simulink model "MSE452_Lab4_grid_side_VOC_student"  (R2023a)
settings: Solver=ode23tb  StartTime=0.0  StopTime=1  MaxStep=1e-5  RelTol=1e-5  AbsTol=1e-5  EnableMultiTasking=on
values from neighbouring files (symbols this model uses):
  Cdc = 4*Cb    [MSE452_Lab4_grid_side_VOC.m]
  Fb = 60    [MSE452_Lab4_grid_side_VOC.m]
  Fs = 2040    [MSE452_Lab4_grid_side_VOC.m]
  Fsampling = 10e3    (= 10000)    [MSE452_Lab4_grid_side_VOC.m]
  Ib = Pb/(Vb)    [MSE452_Lab4_grid_side_VOC.m]
  Lgrid = Lgrid_pu*Lb    [MSE452_Lab4_grid_side_VOC.m]
  Lgrid_pu = 0.2    [MSE452_Lab4_grid_side_VOC.m]
  Rdc_series = 0.1*Zb    [MSE452_Lab4_grid_side_VOC.m]
  Rgrid = Rgrid_pu*Zb    [MSE452_Lab4_grid_side_VOC.m]
  Vb = 690/sqrt(3)    [MSE452_Lab4_grid_side_VOC.m]
  Vdc_ref = sqrt(6)*(1/0.8)    [MSE452_Lab4_grid_side_VOC.m]
  Vdc_supply = Vdc_ref*Vb + Idc*Rdc_series    [MSE452_Lab4_grid_side_VOC.m]
undefined symbols (not defined in the file or in its folder): Rdc
libraries: spsVoltageMeasurementLib x4, spsCurrentMeasurementLib x3, powerlib_extras x3, simulink x3, spsSeriesRLCBranchLib x2, spsControlledVoltageSourceLib x2, simulink_extras x2, spsDCVoltageSourceLib x1, spsUniversalBridgeLib x1, spsThreePhaseSeriesRLCBranchLib x1, spsPower3phInstantaneousLib x1, sps_lib x1
settings Model: Creator=lang  LastModifiedBy=auamai
settings SolverCC: AutoScaleAbsTol=off  AlgebraicLoopSolver=TrustRegion
settings DataIOCC: LimitDataPoints=on  SaveFormat=Array  SignalLoggingSaveFormat=ModelDataLogs  ReturnWorkspaceOutputs=off
settings OptimizationCC: ExpressionDepthLimit=2147483647  InitFltsAndDblsToZero=on  LifeSpan=inf
settings DebuggingCC: SaveWithParameterizedLinksMsg=none  UnderspecifiedInitializationDetection=Classic  MergeDetectMultiDrivingBlocksExec=none  SolverPrmCheckMsg=warning  MultiTaskCondExecSysMsg=none  FcnCallInpInsideContextMsg=warning  UnconnectedInputMsg=warning  UnconnectedOutputMsg=warning  UnconnectedLineMsg=warning  StateNameClashWarn=warning  SFUnexpectedBacktrackingDiag=warning  SFNoUnconditionalDefaultTransitionDiag=warning  SFExecutionAtInitializationDiag=none  ArithmeticOperatorsInVariantConditions=warning
settings HardwareCC: ProdBitPerPointer=32  ProdBitPerSizeT=32  ProdBitPerPtrDiffT=32  ProdLargestAtomicFloat=None  ProdIntDivRoundTo=Undefined  ProdEndianess=Unspecified  ProdWordSize=32  ProdHWDeviceType=32-bit Generic
settings ModelReferenceCC: EnableRefExpFcnMdlSchedulingChecks=on  PropagateSignalLabelsOutOfModel=off
settings SFSimCC: SimUseLocalCustomCode=off  SimParseCustomCode=off  CustomCodeUndefinedFunction=UseInterfaceOnly
settings RTWCC: RTWUseLocalCustomCode=off
settings CodeAppCC: StateflowObjectComments=on
settings GRTTargetCC: TargetFcnLib=ansi_tfl_tmw.mat  TargetLangStandard=C89/C90 (ANSI)  CombineOutputUpdateFcns=off  GRTInterface=on
settings ConfigComp: CovMetricSettings=dw  CovSaveCumulativeToWorkspaceVar=on  CovSaveSingleToWorkspaceVar=on  CovExternalEMLEnable=off
settings SimscapeCC: SimscapeNormalizeSystem=off

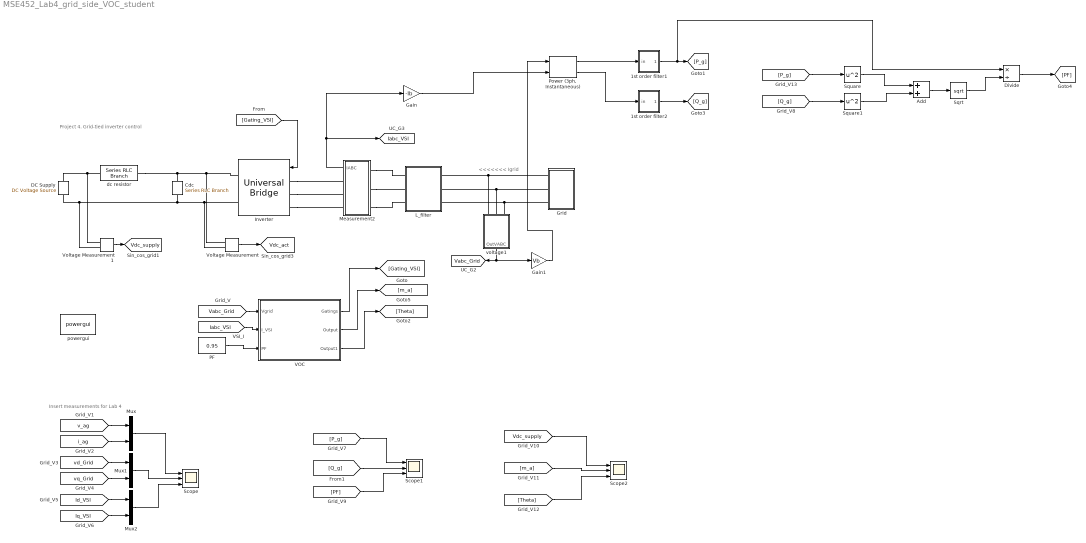
== system MSE452_Lab4_grid_side_VOC_student ==
  note: Insert measurements for Lab 4
  note: <<<<<<< Igrid
  note: Project 4. Grid-tied inverter control
  " voltage1" : Subsystem  mask{Base=Vb}
      mask prompts: Base "Base value"
  1st order filter1 : Subsystem  mask{F0=10, Fs=Fsampling}
      mask prompts: F0 "Cut off Frequency"; Fs "Sampling Frequency"
  1st order filter2 : Subsystem  mask{F0=10, Fs=Fsampling}
      mask prompts: F0 "Cut off Frequency"; Fs "Sampling Frequency"
  Add : Sum
  Cdc : spsSeriesRLCBranchLib/Series RLC Branch  LConnTagsString=__new0  RConnTagsString=__new0  BranchType=C  Resistance=Rdc  Inductance=1e-3  SetiL0=off  InitialCurrent=0  Capacitance=Cdc  Setx0=on  InitialVoltage=Vdc_capacitor_initial  Measurements=None
  DC Supply : spsDCVoltageSourceLib/DC Voltage Source  Amplitude=Vdc_supply*1.0  Measurements=None
  Divide : Product  Inputs=*/
  Gain : Gain  Gain=-Ib
  Gain1 : Gain  Gain=Vb
  Grid : Subsystem
  Inverter : spsUniversalBridgeLib/Universal Bridge  Arms=3  SnubberResistance=1e5  SnubberCapacitance=inf  Device=IGBT / Diodes  Ron=1e-6  Lon=0  ForwardVoltages="[  0  0  ]"  ForwardVoltage=0  GTOparameters=[ 10e-6 , 20e-6 ]  IGBTparameters=[ 1e-6 , 2e-6 ]  Measurements=None  Measurements_2=None  converterType=Rectifier
  L_filter : Subsystem
  Measurement2 : Subsystem  mask{Base=Ib}
      mask prompts: Base "Base value"
  Mux : Mux  Inputs=2
  Mux1 : Mux  Inputs=2
  Mux2 : Mux  Inputs=2
  PF : Constant  Value=0.95
  "Power (3ph, Instantaneous)" : spsPower3phInstantaneousLib/Power (3ph, Instantaneous)
  Scope : Scope  NumInputPorts=3
  Scope1 : Scope  NumInputPorts=3
  Scope2 : Scope  NumInputPorts=3
  Sqrt : Sqrt
  Square : Math  Operator=square
  Square1 : Math  Operator=square
  VOC : Subsystem
  Voltage Measurement : spsVoltageMeasurementLib/Voltage Measurement  PhasorSimulation=off  OutputType=Complex  PSBequivalent=0
  Voltage Measurement1 : spsVoltageMeasurementLib/Voltage Measurement  PhasorSimulation=off  OutputType=Complex  PSBequivalent=0
  dc resistor : spsSeriesRLCBranchLib/Series RLC Branch  LConnTagsString=__new0  RConnTagsString=__new0  BranchType=R  Resistance=Rdc_series  Inductance=1e-3  SetiL0=off  InitialCurrent=0  Capacitance=1e-6  Setx0=off  InitialVoltage=0  Measurements=None
  powergui : sps_lib/powergui  Priority=1  SimulationMode=Continuous  SampleTime=50e-6  frequency=60  Iterations=50  frequencyindice=0  Pbase=100e6  ErrMax=1e-4  UnitsV=kV  UnitsW=MW  buscounter=0  FunctionMessages=off  echomessages=off  EnableUseOfTLC=off  CurrentSourceSwitches=on  DisableSnubberDevices=off  DisableRonSwitches=off  DisableVfSwitches=off  DisplayEquations=off  AutomaticDiscreteSolvers=off  SolverType=Tustin  Interpol=off  ExternalGateDelay=off  methode=off  Ts=100  x0status=blocks  SPID=off  SwTol=0  HookPort=off  NonlinearTolerance=1e-4  nMaxIteration=100  ContinueOnMaxIteration=off  RestoreLinks=warning  ResistiveCurrentMeasurement=off  Frange=[0:2:500]  Ylog=off  Xlog=on  ShowGrid=off  save=off  variable=ZData  structure=0  ZoomFFT=off  StartTime=0.0  cycles=1  DisplayStyle=1  fundamental=60  FreqAxis=off  MaxFrequency=1000  frequencyindicesteady=1  RmsSteady=1  display=off
  tag scope: Iabc_VSI=global, Vabc_Grid=global, Vdc_act=global, Vdc_supply=global
  wires:
  [Vabc_Grid] -> VOC/1(Vgrid)
  [Iabc_VSI] -> VOC/2(I_VSI)
  VOC/1(Gatings) -> [Gating_VSI]
  [Gating_VSI] -> Inverter/1
  Voltage Measurement/1 -> [Vdc_act]
  Voltage Measurement1/1 -> [Vdc_supply]
  Measurement2/1(IABC) -> Gain/1, [Iabc_VSI]
  " voltage1"/1(OutVABC) -> Gain1/1, [Vabc_Grid]
  [v_ag] -> Mux/1
  [i_ag] -> Mux/2
  [vq_Grid] -> Mux1/2
  [vd_Grid] -> Mux1/1
  [Id_VSI] -> Mux2/1
  [Iq_VSI] -> Mux2/2
  PF/1 -> VOC/3(PF)
  Mux/1 -> Scope/1
  Mux1/1 -> Scope/2
  Mux2/1 -> Scope/3
  [P_g] -> Scope1/1
  [Q_g] -> Scope1/2
  [PF] -> Scope1/3
  [Vdc_supply] -> Scope2/1
  [m_a] -> Scope2/2
  [Theta] -> Scope2/3
  VOC/2(Output) -> [m_a]
  VOC/3(Output1) -> [Theta]
  Gain/1 -> "Power (3ph, Instantaneous)"/2
  Gain1/1 -> "Power (3ph, Instantaneous)"/1
  "Power (3ph, Instantaneous)"/1 -> 1st order filter1/1(in)
  "Power (3ph, Instantaneous)"/2 -> 1st order filter2/1(in)
  1st order filter1/1(Out) -> Divide/1, [P_g]
  1st order filter2/1(Out) -> [Q_g]
  [P_g] -> Square/1
  [Q_g] -> Square1/1
  Square/1 -> Add/1
  Square1/1 -> Add/2
  Add/1 -> Sqrt/1
  Sqrt/1 -> Divide/2
  Divide/1 -> [PF]
  connections:
  Cdc/RConn1 -- Voltage Measurement/LConn1 -- Inverter/RConn1 -- dc resistor/RConn1
  Inverter/RConn2 -- Voltage Measurement/LConn2 -- Cdc/LConn1 -- DC Supply/LConn1 -- Voltage Measurement1/LConn2
  DC Supply/RConn1 -- dc resistor/LConn1 -- Voltage Measurement1/LConn1
  Inverter/LConn1 -- Measurement2/RConn1
  Inverter/LConn2 -- Measurement2/RConn2
  Inverter/LConn3 -- Measurement2/RConn3
  Measurement2/LConn1 -- L_filter/RConn1
  Measurement2/LConn2 -- L_filter/RConn2
  Measurement2/LConn3 -- L_filter/RConn3
  " voltage1"/LConn1 -- Grid/RConn1 -- L_filter/LConn1
  " voltage1"/LConn2 -- Grid/RConn2 -- L_filter/LConn2
  " voltage1"/LConn3 -- Grid/RConn3 -- L_filter/LConn3

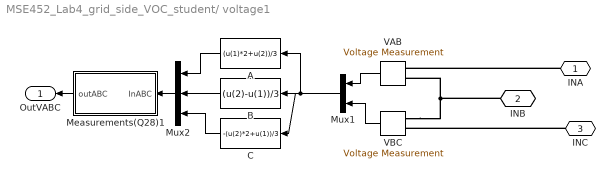
== system MSE452_Lab4_grid_side_VOC_student/ voltage1 ==
  A : Fcn  Expr=(u(1)*2+u(2))/3
  B : Fcn  Expr=(u(2)-u(1))/3
  C : Fcn  Expr=-(u(2)*2+u(1))/3
  Measurements(Q28)1 : Subsystem  mask{Base=Base}
      mask prompts: Base "Base Value"
  Mux1 : Mux  Inputs=2
  Mux2 : Mux  Inputs=3
  VAB : spsVoltageMeasurementLib/Voltage Measurement  PhasorSimulation=off  OutputType=Complex  PSBequivalent=0
  VBC : spsVoltageMeasurementLib/Voltage Measurement  PhasorSimulation=off  OutputType=Complex  PSBequivalent=0
  INA : PMIOPort  Side=Left
  INB : PMIOPort  Port=2  Side=Left
  INC : PMIOPort  Port=3  Side=Left
  OutVABC : Outport
  wires:
  Measurements(Q28)1/1(outABC) -> OutVABC/1
  VAB/1 -> Mux1/1
  VBC/1 -> Mux1/2
  Mux1/1 -> A/1, B/1, C/1
  A/1 -> Mux2/1
  B/1 -> Mux2/2
  Mux2/1 -> Measurements(Q28)1/1(InABC)
  C/1 -> Mux2/3
  connections:
  VBC/LConn1 -- VAB/LConn2 -- INB/RConn1
  INC/RConn1 -- VBC/LConn2
  INA/RConn1 -- VAB/LConn1

== system MSE452_Lab4_grid_side_VOC_student/1st order filter1 ==
  in : Inport
  Discrete Transfer 1Hz3 : DiscreteTransferFcn  Numerator=[1/Fs*(2*pi*F0) 1/Fs*(2*pi*F0) ]  Denominator="[((2*pi*F0)/Fs+2)  ((2*pi*F0)/Fs-2)]"  SampleTime=1/Fs
  Out : Outport
  wires:
  in/1 -> Discrete Transfer 1Hz3/1
  Discrete Transfer 1Hz3/1 -> Out/1

== system MSE452_Lab4_grid_side_VOC_student/1st order filter2 ==
  in : Inport
  Discrete Transfer 1Hz3 : DiscreteTransferFcn  Numerator=[1/Fs*(2*pi*F0) 1/Fs*(2*pi*F0) ]  Denominator="[((2*pi*F0)/Fs+2)  ((2*pi*F0)/Fs-2)]"  SampleTime=1/Fs
  Out : Outport
  wires:
  Discrete Transfer 1Hz3/1 -> Out/1
  in/1 -> Discrete Transfer 1Hz3/1

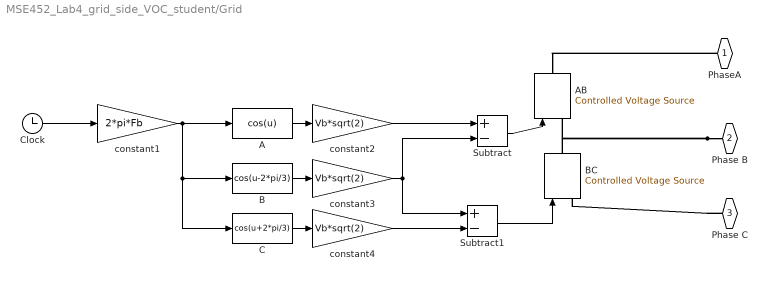
== system MSE452_Lab4_grid_side_VOC_student/Grid ==
  A : Fcn  Expr=cos(u)
  AB : spsControlledVoltageSourceLib/Controlled Voltage Source  Initialize=off  Source_Type=AC  Amplitude=0  Phase=0  Frequency=0  Measurements=None
  B : Fcn  Expr=cos(u-2*pi/3)
  BC : spsControlledVoltageSourceLib/Controlled Voltage Source  Initialize=off  Source_Type=AC  Amplitude=0  Phase=0  Frequency=0  Measurements=None
  C : Fcn  Expr=cos(u+2*pi/3)
  Clock : Clock
  Subtract : Sum  Inputs=+-
  Subtract1 : Sum  Inputs=+-
  constant1 : Gain  Gain=2*pi*Fb
  constant2 : Gain  Gain=Vb*sqrt(2)
  constant3 : Gain  Gain=Vb*sqrt(2)
  constant4 : Gain  Gain=Vb*sqrt(2)
  PhaseA : PMIOPort  Side=Right
  Phase B : PMIOPort  Port=2  Side=Right
  Phase C : PMIOPort  Port=3  Side=Right
  wires:
  Subtract/1 -> AB/1
  Subtract1/1 -> BC/1
  A/1 -> constant2/1
  B/1 -> constant3/1
  C/1 -> constant4/1
  Clock/1 -> constant1/1
  constant1/1 -> A/1, B/1, C/1
  constant2/1 -> Subtract/1
  constant3/1 -> Subtract/2, Subtract1/1
  constant4/1 -> Subtract1/2
  connections:
  Phase B/RConn1 -- BC/RConn1 -- AB/LConn1
  PhaseA/RConn1 -- AB/RConn1
  Phase C/RConn1 -- BC/LConn1

== system MSE452_Lab4_grid_side_VOC_student/L_filter ==
  Three-Phase Series RLC Branch1 : spsThreePhaseSeriesRLCBranchLib/Three-Phase Series RLC Branch  LConnTagsString=A|B|C  RConnTagsString=A|B|C  BranchType=RL  Resistance=Rgrid  Inductance=Lgrid  Capacitance=1e-6  Measurements=None
  In_A : PMIOPort  Side=Left
  out_A : PMIOPort  Port=2  Side=Right
  In_B : PMIOPort  Port=3  Side=Left
  out_B : PMIOPort  Port=4  Side=Right
  In_C : PMIOPort  Port=5  Side=Left
  out_C : PMIOPort  Port=6  Side=Right
  connections:
  In_B/RConn1 -- Three-Phase Series RLC Branch1/LConn2
  out_C/RConn1 -- Three-Phase Series RLC Branch1/RConn3
  out_B/RConn1 -- Three-Phase Series RLC Branch1/RConn2
  out_A/RConn1 -- Three-Phase Series RLC Branch1/RConn1
  Three-Phase Series RLC Branch1/LConn1 -- In_A/RConn1
  Three-Phase Series RLC Branch1/LConn3 -- In_C/RConn1

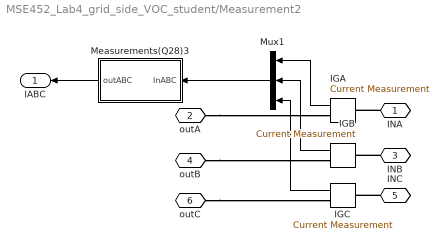
== system MSE452_Lab4_grid_side_VOC_student/Measurement2 ==
  IGA : spsCurrentMeasurementLib/Current Measurement  PhasorSimulation=off  OutputType=Complex  PSBequivalent=0
  IGB : spsCurrentMeasurementLib/Current Measurement  PhasorSimulation=off  OutputType=Complex  PSBequivalent=0
  IGC : spsCurrentMeasurementLib/Current Measurement  PhasorSimulation=off  OutputType=Complex  PSBequivalent=0
  Measurements(Q28)3 : Subsystem  mask{Base=Base}
      mask prompts: Base "Base Value"
  Mux1 : Mux  Inputs=3
  INA : PMIOPort  Side=Left
  outA : PMIOPort  Port=2  Side=Right
  INB : PMIOPort  Port=3  Side=Left
  outB : PMIOPort  Port=4  Side=Right
  INC : PMIOPort  Port=5  Side=Left
  outC : PMIOPort  Port=6  Side=Right
  IABC : Outport
  wires:
  Measurements(Q28)3/1(outABC) -> IABC/1
  Mux1/1 -> Measurements(Q28)3/1(InABC)
  IGA/1 -> Mux1/1
  IGB/1 -> Mux1/2
  IGC/1 -> Mux1/3
  connections:
  outC/RConn1 -- IGC/RConn1
  INC/RConn1 -- IGC/LConn1
  outB/RConn1 -- IGB/RConn1
  INB/RConn1 -- IGB/LConn1
  outA/RConn1 -- IGA/RConn1
  INA/RConn1 -- IGA/LConn1

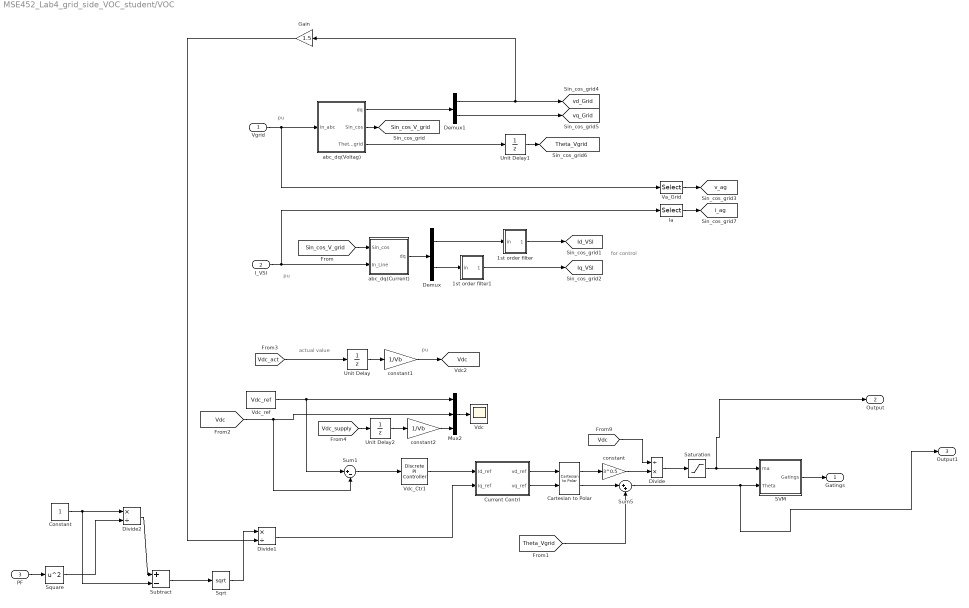
== system MSE452_Lab4_grid_side_VOC_student/VOC ==
  note: for control
  note: pu
  note: pu
  note: actual value
  note: pu
  Vgrid : Inport
  I_VSI : Inport  Port=2
  PF : Inport  Port=3
  1st order filter : Subsystem  mask{F0=500, Fs=Fsampling}
      mask prompts: F0 "Cut off Frequency"; Fs "Sampling Frequency"
  1st order filter1 : Subsystem  mask{F0=500, Fs=Fsampling}
      mask prompts: F0 "Cut off Frequency"; Fs "Sampling Frequency"
  Cartesian to Polar : simulink_extras/Transformations/Cartesian to Polar
  Constant : Constant
  Current Contrl : Subsystem
  Demux : Demux  Outputs=2
  Demux1 : Demux  Outputs=2
  Divide : Product  Inputs=/*
  Divide1 : Product  Inputs=*/
  Divide2 : Product  Inputs=*/
  Gain : Gain  Gain=1.5
  Ia : Selector  InputPortWidth=3  IndexOptions=Index vector (dialog)  Indices=1  OutputSizes=1
  Mux2 : Mux  Inputs=3
  SVM : Subsystem  mask{Fs=Fs}
      mask prompts: Fs "Switching frequency"
  Saturation : Saturate  UpperLimit=1  LowerLimit=0  SampleTime=1/Fsampling
  Sqrt : Sqrt
  Square : Math  Operator=square
  Subtract : Sum  Inputs=+-
  Sum1 : Sum  Inputs=|+-
  Sum5 : Sum  Inputs=|++
  Unit Delay : UnitDelay  InitialCondition=Vb*3^0.5  SampleTime=1/Fsampling  HasFrameUpgradeWarning=on
  Unit Delay1 : UnitDelay  InitialCondition=Vb*3^0.5  SampleTime=1/Fsampling  HasFrameUpgradeWarning=on
  Unit Delay2 : UnitDelay  InitialCondition=Vb*3^0.5  SampleTime=1/Fsampling  HasFrameUpgradeWarning=on
  Va_Grid : Selector  InputPortWidth=3  IndexOptions=Index vector (dialog)  Indices=1  OutputSizes=1
  Vdc : Scope
  Vdc_Ctr1 : powerlib_extras/Discrete  Control Blocks/Discrete PI Controller  Kp=1.0  Ki=200  Par_Limits=[1.5 -1.5]  Init=0  Ts=1/Fsampling
  Vdc_ref : Constant  Value=Vdc_ref
  abc_dq(Current) : Subsystem
  abc_dq(Voltag) : Subsystem
  constant : Gain  Gain=3^0.5
  constant1 : Gain  Gain=1/Vb
  constant2 : Gain  Gain=1/Vb
  Gatings : Outport
  Output : Outport  Port=2
  Output1 : Outport  Port=3
  tag scope: Id_VSI=global, Iq_VSI=global, Sin_cos_V_grid=global, Theta_Vgrid=global, Vdc=global, i_ag=global, v_ag=global, vd_Grid=global, vq_Grid=global
  wires:
  abc_dq(Current)/1(dq) -> Demux/1
  abc_dq(Voltag)/1(dq) -> Demux1/1
  Vgrid/1 -> abc_dq(Voltag)/1(In_abc), Va_Grid/1
  abc_dq(Voltag)/2(Sin_cos) -> [Sin_cos_V_grid]
  [Sin_cos_V_grid] -> abc_dq(Current)/1(Sin_cos)
  I_VSI/1 -> abc_dq(Current)/2(In_Line), Ia/1
  Demux/1 -> 1st order filter/1(in)
  Demux/2 -> 1st order filter1/1(in)
  Demux1/1 -> Gain/1, [vd_Grid]
  Demux1/2 -> [vq_Grid]
  abc_dq(Voltag)/3(Theta_Vgrid) -> Unit Delay1/1
  [Vdc_act] -> Unit Delay/1
  constant1/1 -> [Vdc]
  Cartesian to Polar/1 -> constant/1
  Cartesian to Polar/2 -> Sum5/1
  Current Contrl/1(vd_ref) -> Cartesian to Polar/1
  Current Contrl/2(vq_ref) -> Cartesian to Polar/2
  [Vdc] -> Divide/1
  constant/1 -> Divide/2
  Divide/1 -> Saturation/1
  [Vdc] -> Sum1/2, Mux2/2
  Sum1/1 -> Vdc_Ctr1/1
  1st order filter/1(Out) -> [Id_VSI]
  1st order filter1/1(Out) -> [Iq_VSI]
  SVM/1(Gatings) -> Gatings/1
  Vdc_ref/1 -> Sum1/1, Mux2/1
  Unit Delay/1 -> constant1/1
  Vdc_Ctr1/1 -> Current Contrl/1(Id_ref)
  Mux2/1 -> Vdc/1
  [Theta_Vgrid] -> Sum5/2
  Unit Delay1/1 -> [Theta_Vgrid]
  Unit Delay2/1 -> constant2/1
  constant2/1 -> Mux2/3
  [Vdc_supply] -> Unit Delay2/1
  Saturation/1 -> Output/1, SVM/1(ma)
  Va_Grid/1 -> [v_ag]
  Ia/1 -> [i_ag]
  Gain/1 -> Divide1/2
  Divide1/1 -> Current Contrl/2(Iq_ref)
  PF/1 -> Square/1
  Constant/1 -> Subtract/2, Divide2/1
  Square/1 -> Divide2/2
  Divide2/1 -> Subtract/1
  Subtract/1 -> Sqrt/1
  Sqrt/1 -> Divide1/1
  Sum5/1 -> Output1/1, SVM/2(Theta)

== system MSE452_Lab4_grid_side_VOC_student/ voltage1/Measurements(Q28)1 ==
  InABC : Inport
  Demux : Demux  Outputs=3
  Gain1 : Gain  Gain=1/Base
  Gain2 : Gain  Gain=1/Base
  Gain3 : Gain  Gain=1/Base
  Mux : Mux  Inputs=3
  outABC : Outport
  wires:
  Mux/1 -> outABC/1
  Demux/1 -> Gain2/1
  InABC/1 -> Demux/1
  Gain2/1 -> Mux/1
  Gain1/1 -> Mux/2
  Gain3/1 -> Mux/3
  Demux/2 -> Gain1/1
  Demux/3 -> Gain3/1

== system MSE452_Lab4_grid_side_VOC_student/Measurement2/Measurements(Q28)3 ==
  InABC : Inport
  Demux : Demux  Outputs=3
  Gain1 : Gain  Gain=1/Base
  Gain2 : Gain  Gain=1/Base
  Gain3 : Gain  Gain=1/Base
  Mux : Mux  Inputs=3
  outABC : Outport
  wires:
  Mux/1 -> outABC/1
  Demux/1 -> Gain2/1
  InABC/1 -> Demux/1
  Gain2/1 -> Mux/1
  Gain1/1 -> Mux/2
  Gain3/1 -> Mux/3
  Demux/2 -> Gain1/1
  Demux/3 -> Gain3/1

== system MSE452_Lab4_grid_side_VOC_student/VOC/1st order filter ==
  in : Inport
  Discrete Transfer 1Hz3 : DiscreteTransferFcn  Numerator=[1/Fs*(2*pi*F0) 1/Fs*(2*pi*F0) ]  Denominator="[((2*pi*F0)/Fs+2)  ((2*pi*F0)/Fs-2)]"  SampleTime=1/Fs
  Out : Outport
  wires:
  Discrete Transfer 1Hz3/1 -> Out/1
  in/1 -> Discrete Transfer 1Hz3/1

== system MSE452_Lab4_grid_side_VOC_student/VOC/1st order filter1 ==
  in : Inport
  Discrete Transfer 1Hz3 : DiscreteTransferFcn  Numerator=[1/Fs*(2*pi*F0) 1/Fs*(2*pi*F0) ]  Denominator="[((2*pi*F0)/Fs+2)  ((2*pi*F0)/Fs-2)]"  SampleTime=1/Fs
  Out : Outport
  wires:
  in/1 -> Discrete Transfer 1Hz3/1
  Discrete Transfer 1Hz3/1 -> Out/1

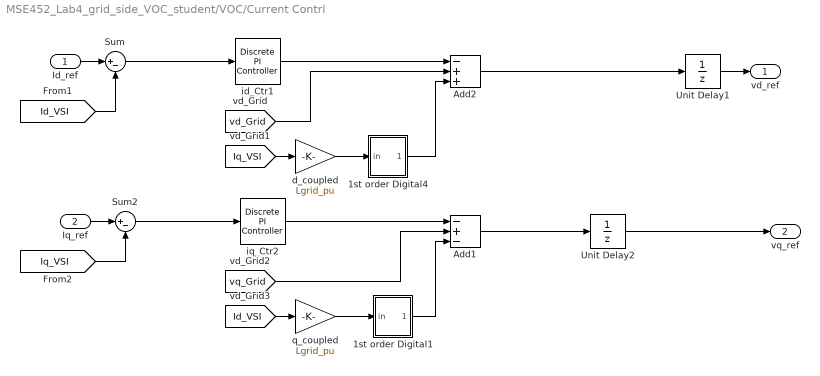
== system MSE452_Lab4_grid_side_VOC_student/VOC/Current Contrl ==
  Id_ref : Inport
  Iq_ref : Inport  Port=2
  1st order Digital1 : Subsystem  mask{F0=10, Fs=Fsampling}
      mask prompts: F0 "Cut off Frequency"; Fs "Sampling Frequency"
  1st order Digital4 : Subsystem  mask{F0=10, Fs=Fsampling}
      mask prompts: F0 "Cut off Frequency"; Fs "Sampling Frequency"
  Add1 : Sum  Inputs=-+-
  Add2 : Sum  Inputs=-++
  Sum : Sum  Inputs=|+-
  Sum2 : Sum  Inputs=|+-
  Unit Delay1 : UnitDelay  SampleTime=1/Fsampling  HasFrameUpgradeWarning=on
  Unit Delay2 : UnitDelay  SampleTime=1/Fsampling  HasFrameUpgradeWarning=on
  d_coupled : Gain  Gain=Lgrid_pu
  id_Ctr1 : powerlib_extras/Discrete  Control Blocks/Discrete PI Controller  Kp=0.3  Ki=200  Par_Limits=[1 -1]  Init=0  Ts=1/Fsampling
  iq_Ctr2 : powerlib_extras/Discrete  Control Blocks/Discrete PI Controller  Kp=0.3  Ki=200  Par_Limits=[1 -1]  Init=0  Ts=1/Fsampling
  q_coupled : Gain  Gain=Lgrid_pu
  vd_ref : Outport
  vq_ref : Outport  Port=2
  wires:
  id_Ctr1/1 -> Add2/1
  [vd_Grid] -> Add2/2
  [Iq_VSI] -> d_coupled/1
  Sum/1 -> id_Ctr1/1
  iq_Ctr2/1 -> Add1/1
  [vq_Grid] -> Add1/2
  [Id_VSI] -> q_coupled/1
  Sum2/1 -> iq_Ctr2/1
  [Id_VSI] -> Sum/2
  [Iq_VSI] -> Sum2/2
  Id_ref/1 -> Sum/1
  Add2/1 -> Unit Delay1/1
  Iq_ref/1 -> Sum2/1
  Add1/1 -> Unit Delay2/1
  d_coupled/1 -> 1st order Digital4/1(in)
  q_coupled/1 -> 1st order Digital1/1(in)
  1st order Digital4/1(Out) -> Add2/3
  1st order Digital1/1(Out) -> Add1/3
  Unit Delay2/1 -> vq_ref/1
  Unit Delay1/1 -> vd_ref/1

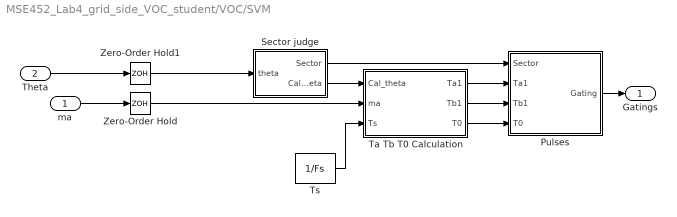
== system MSE452_Lab4_grid_side_VOC_student/VOC/SVM ==
  ma : Inport
  Theta : Inport  Port=2
  Pulses : Subsystem
  Sector judge : Subsystem
  Ta Tb T0 Calculation : Subsystem
  Ts : Constant  Value=1/Fs
  Zero-Order Hold : ZeroOrderHold  SampleTime=1/(2*Fs)
  Zero-Order Hold1 : ZeroOrderHold  SampleTime=1/(2*Fs)
  Gatings : Outport
  wires:
  Ta Tb T0 Calculation/3(T0) -> Pulses/4(T0)
  Ts/1 -> Ta Tb T0 Calculation/3(Ts)
  Ta Tb T0 Calculation/1(Ta1) -> Pulses/2(Ta1)
  Ta Tb T0 Calculation/2(Tb1) -> Pulses/3(Tb1)
  Sector judge/1(Sector) -> Pulses/1(Sector)
  Sector judge/2(Cal_theta) -> Ta Tb T0 Calculation/1(Cal_theta)
  Theta/1 -> Zero-Order Hold1/1
  Pulses/1(Gating) -> Gatings/1
  ma/1 -> Zero-Order Hold/1
  Zero-Order Hold/1 -> Ta Tb T0 Calculation/2(ma)
  Zero-Order Hold1/1 -> Sector judge/1(theta)

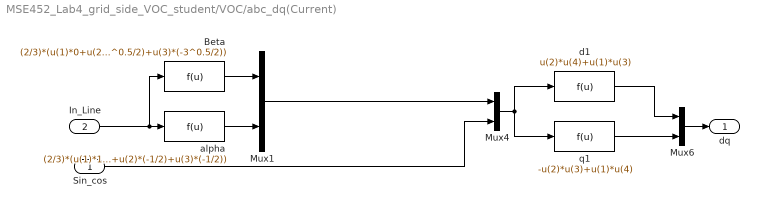
== system MSE452_Lab4_grid_side_VOC_student/VOC/abc_dq(Current) ==
  Sin_cos : Inport
  In_Line : Inport  Port=2
  Beta : Fcn  Expr=(2/3)*(u(1)*0+u(2)*(3^0.5/2)+u(3)*(-3^0.5/2))
  Mux1 : Mux  Inputs=2
  Mux4 : Mux  Inputs=2
  Mux6 : Mux  Inputs=2
  alpha : Fcn  Expr=(2/3)*(u(1)*1+u(2)*(-1/2)+u(3)*(-1/2))
  d1 : Fcn  Expr=u(2)*u(4)+u(1)*u(3)
  q1 : Fcn  Expr=-u(2)*u(3)+u(1)*u(4)
  dq : Outport
  wires:
  Sin_cos/1 -> Mux4/2
  Beta/1 -> Mux1/1
  alpha/1 -> Mux1/2
  Mux1/1 -> Mux4/1
  In_Line/1 -> Beta/1, alpha/1
  Mux4/1 -> q1/1, d1/1
  d1/1 -> Mux6/1
  q1/1 -> Mux6/2
  Mux6/1 -> dq/1

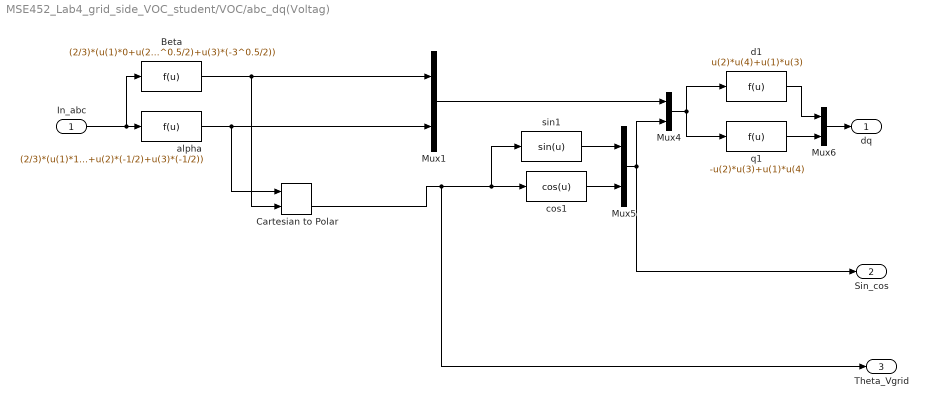
== system MSE452_Lab4_grid_side_VOC_student/VOC/abc_dq(Voltag) ==
  In_abc : Inport
  Beta : Fcn  Expr=(2/3)*(u(1)*0+u(2)*(3^0.5/2)+u(3)*(-3^0.5/2))
  Cartesian to Polar : simulink_extras/Transformations/Cartesian to Polar
  Mux{1,4..6} (4 alike) : Mux  Inputs=2
  alpha : Fcn  Expr=(2/3)*(u(1)*1+u(2)*(-1/2)+u(3)*(-1/2))
  cos1 : Fcn  Expr=cos(u)
  d1 : Fcn  Expr=u(2)*u(4)+u(1)*u(3)
  q1 : Fcn  Expr=-u(2)*u(3)+u(1)*u(4)
  sin1 : Fcn  Expr=sin(u)
  dq : Outport
  Sin_cos : Outport  Port=2
  Theta_Vgrid : Outport  Port=3
  wires:
  Mux6/1 -> dq/1
  q1/1 -> Mux6/2
  d1/1 -> Mux6/1
  cos1/1 -> Mux5/2
  sin1/1 -> Mux5/1
  Mux4/1 -> d1/1, q1/1
  In_abc/1 -> alpha/1, Beta/1
  Mux1/1 -> Mux4/1
  alpha/1 -> Cartesian to Polar/1, Mux1/2
  Beta/1 -> Cartesian to Polar/2, Mux1/1
  Mux5/1 -> Mux4/2, Sin_cos/1
  Cartesian to Polar/2 -> cos1/1, sin1/1, Theta_Vgrid/1

== system MSE452_Lab4_grid_side_VOC_student/VOC/Current Contrl/1st order Digital1 ==
  in : Inport
  Discrete Transfer 1Hz3 : DiscreteTransferFcn  Numerator=[1/Fs*(2*pi*F0) 1/Fs*(2*pi*F0) ]  Denominator="[((2*pi*F0)/Fs+2)  ((2*pi*F0)/Fs-2)]"  SampleTime=1/Fs
  Out : Outport
  wires:
  in/1 -> Discrete Transfer 1Hz3/1
  Discrete Transfer 1Hz3/1 -> Out/1

== system MSE452_Lab4_grid_side_VOC_student/VOC/Current Contrl/1st order Digital4 ==
  in : Inport
  Discrete Transfer 1Hz3 : DiscreteTransferFcn  Numerator=[1/Fs*(2*pi*F0) 1/Fs*(2*pi*F0) ]  Denominator="[((2*pi*F0)/Fs+2)  ((2*pi*F0)/Fs-2)]"  SampleTime=1/Fs
  Out : Outport
  wires:
  Discrete Transfer 1Hz3/1 -> Out/1
  in/1 -> Discrete Transfer 1Hz3/1

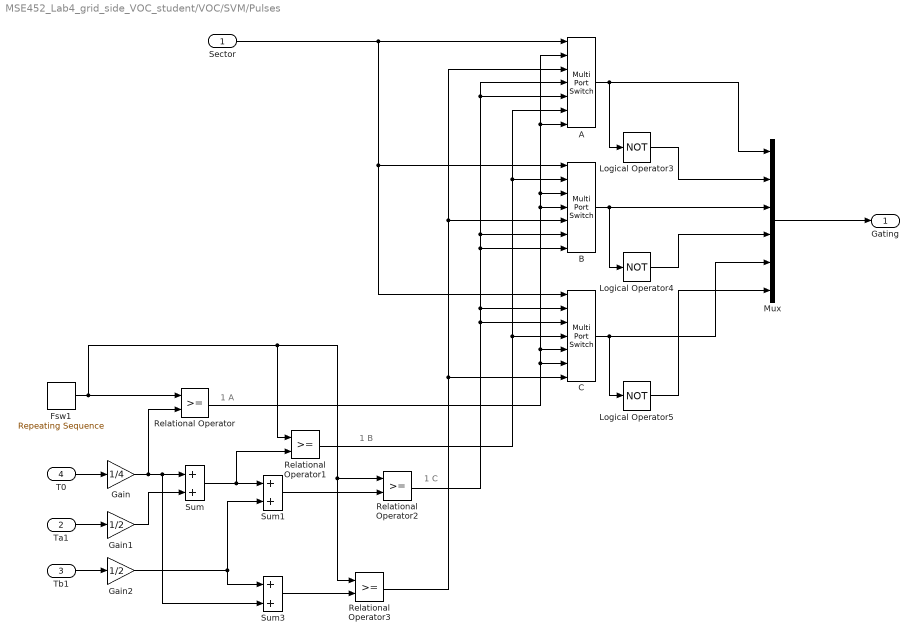
== system MSE452_Lab4_grid_side_VOC_student/VOC/SVM/Pulses ==
  note: 1 A
  note: 1 B
  note: 1 C
  Sector : Inport
  Ta1 : Inport  Port=2
  Tb1 : Inport  Port=3
  T0 : Inport  Port=4
  A : MultiPortSwitch  Inputs=6  SaturateOnIntegerOverflow=off  InputSameDT=off
  B : MultiPortSwitch  Inputs=6  SaturateOnIntegerOverflow=off  InputSameDT=off
  C : MultiPortSwitch  Inputs=6  SaturateOnIntegerOverflow=off  InputSameDT=off
  Fsw1 : simulink/Sources/Repeating Sequence  rep_seq_t=[0 1/Fs/2 1/Fs]  rep_seq_y=[0 1/Fs/2 0]
  Gain : Gain  Gain=1/4
  Gain1 : Gain  Gain=1/2
  Gain2 : Gain  Gain=1/2
  Logical Operator3 : Logic  Operator=NOT  AllPortsSameDT=off
  Logical Operator4 : Logic  Operator=NOT  AllPortsSameDT=off
  Logical Operator5 : Logic  Operator=NOT  AllPortsSameDT=off
  Mux : Mux  Inputs=6
  Relational Operator{,1..3} (4 alike) : RelationalOperator  OutDataTypeStr=boolean  InputSameDT=off
  Sum : Sum
  Sum1 : Sum
  Sum3 : Sum
  Gating : Outport
  wires:
  T0/1 -> Gain/1
  Ta1/1 -> Gain1/1
  Tb1/1 -> Gain2/1
  Gain/1 -> Relational Operator/2, Sum/1, Sum3/2
  Gain1/1 -> Sum/2
  Gain2/1 -> Sum1/2, Sum3/1
  Sum/1 -> Sum1/1, Relational Operator1/2
  Fsw1/1 -> Relational Operator/1, Relational Operator1/1, Relational Operator2/1, Relational Operator3/1
  Sum1/1 -> Relational Operator2/2
  Sector/1 -> A/1, C/1, B/1
  A/1 -> Logical Operator3/1, Mux/1
  B/1 -> Logical Operator4/1, Mux/3
  C/1 -> Logical Operator5/1, Mux/5
  Relational Operator/1 -> A/2, A/7, B/3, B/4, C/5, C/6
  Relational Operator1/1 -> C/4, B/2, A/6
  Relational Operator2/1 -> B/7, A/4, A/5, B/6, C/2, C/3
  Mux/1 -> Gating/1
  Logical Operator3/1 -> Mux/2
  Logical Operator4/1 -> Mux/4
  Logical Operator5/1 -> Mux/6
  Sum3/1 -> Relational Operator3/2
  Relational Operator3/1 -> A/3, B/5, C/7

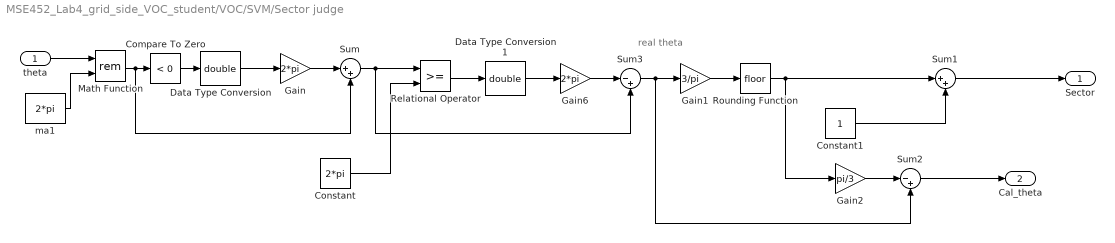
== system MSE452_Lab4_grid_side_VOC_student/VOC/SVM/Sector judge ==
  note: real theta
  theta : Inport
  Compare To Zero : simulink/Logic and Bit Operations/Compare To Zero  relop=<  OutDataTypeStr=uint8  ZeroCross=off
  Constant : Constant  Value=2*pi
  Constant1 : Constant  OutDataTypeStr=boolean
  Data Type Conversion : DataTypeConversion  OutDataTypeStr=double  SaturateOnIntegerOverflow=off  RndMeth=Floor
  Data Type Conversion1 : DataTypeConversion  OutDataTypeStr=double  SaturateOnIntegerOverflow=off  RndMeth=Floor
  Gain : Gain  Gain=2*pi
  Gain1 : Gain  Gain=3/pi
  Gain2 : Gain  Gain=pi/3
  Gain6 : Gain  Gain=2*pi
  Math Function : Math  Operator=rem  SignedPower=on
  Relational Operator : RelationalOperator  OutDataTypeStr=boolean  InputSameDT=off
  Rounding Function : Rounding
  Sum : Sum  Inputs=|++
  Sum1 : Sum  Inputs=|++  SaturateOnIntegerOverflow=on
  Sum2 : Sum  Inputs=|-+
  Sum3 : Sum  Inputs=|-+
  ma1 : Constant  Value=2*pi
  Sector : Outport
  Cal_theta : Outport  Port=2
  wires:
  Math Function/1 -> Compare To Zero/1, Sum/2
  Compare To Zero/1 -> Data Type Conversion/1
  Data Type Conversion/1 -> Gain/1
  Gain/1 -> Sum/1
  Gain1/1 -> Rounding Function/1
  Rounding Function/1 -> Sum1/1, Gain2/1
  Sum1/1 -> Sector/1
  Constant1/1 -> Sum1/2
  Gain2/1 -> Sum2/1
  Sum2/1 -> Cal_theta/1
  Sum/1 -> Relational Operator/1, Sum3/2
  Constant/1 -> Relational Operator/2
  Relational Operator/1 -> Data Type Conversion1/1
  Data Type Conversion1/1 -> Gain6/1
  Gain6/1 -> Sum3/1
  Sum3/1 -> Gain1/1, Sum2/2
  ma1/1 -> Math Function/2
  theta/1 -> Math Function/1

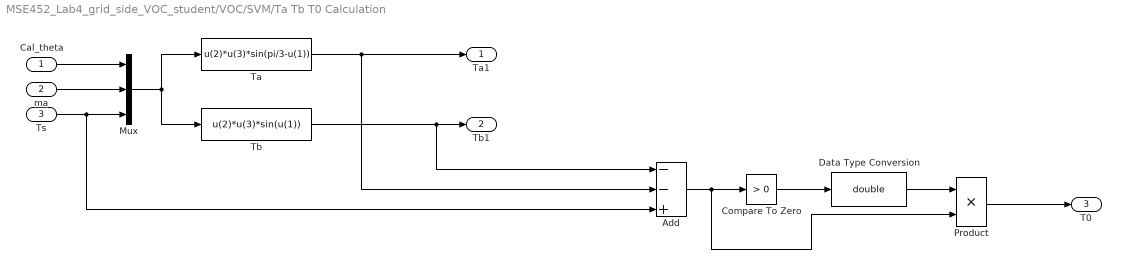
== system MSE452_Lab4_grid_side_VOC_student/VOC/SVM/Ta Tb T0 Calculation ==
  Cal_theta : Inport
  ma : Inport  Port=2
  Ts : Inport  Port=3
  Add : Sum  Inputs=--+
  Compare To Zero : simulink/Logic and Bit Operations/Compare To Zero  relop=>  OutDataTypeStr=boolean
  Data Type Conversion : DataTypeConversion  OutDataTypeStr=double  SaturateOnIntegerOverflow=off  RndMeth=Floor
  Mux : Mux  Inputs=3
  Product : Product  RndMeth=Zero
  Ta : Fcn  Expr=u(2)*u(3)*sin(pi/3-u(1))
  Tb : Fcn  Expr=u(2)*u(3)*sin(u(1))
  Ta1 : Outport
  Tb1 : Outport  Port=2
  T0 : Outport  Port=3
  wires:
  Ts/1 -> Mux/3, Add/3
  ma/1 -> Mux/2
  Cal_theta/1 -> Mux/1
  Mux/1 -> Ta/1, Tb/1
  Ta/1 -> Add/2, Ta1/1
  Product/1 -> T0/1
  Tb/1 -> Tb1/1, Add/1
  Add/1 -> Compare To Zero/1, Product/2
  Compare To Zero/1 -> Data Type Conversion/1
  Data Type Conversion/1 -> Product/1
